simulink model "Controllo_LQ_comp"  (R2023b)
settings: Solver=VariableStepAuto  StartTime=0.0  StopTime=100  RelTol=1e-6
undefined symbols (not defined in the file): A, B, C, Comp, D, K
settings Model: Creator=alfredo  LastModifiedBy=roberto_ambrosino
settings SolverCC: AlgebraicLoopSolver=TrustRegion
settings DataIOCC: ReturnWorkspaceOutputs=off
settings DebuggingCC: UnconnectedInputMsg=warning  UnconnectedOutputMsg=warning  UnconnectedLineMsg=warning  ArithmeticOperatorsInVariantConditions=warning
settings ModelReferenceCC: EnableRefExpFcnMdlSchedulingChecks=on
settings SFSimCC: SimUseLocalCustomCode=off  CustomCodeUndefinedFunction=UseInterfaceOnly
settings RTWCC: RTWUseLocalCustomCode=off

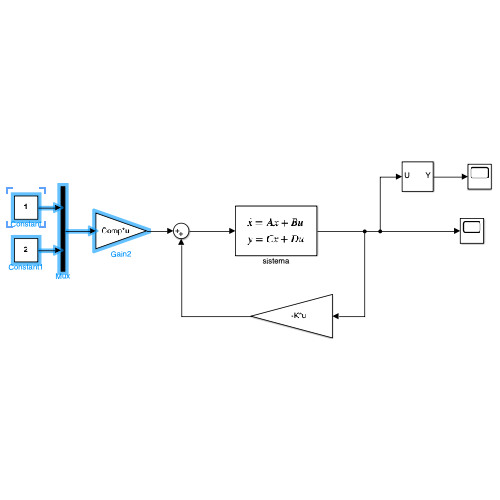
[thumbnail: Simulink's stored preview of the top-level diagram]
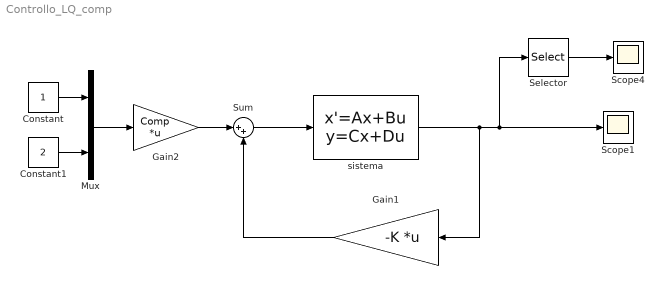
== system Controllo_LQ_comp ==
  Constant : Constant
  Constant1 : Constant  Value=2
  Gain1 : Gain  Gain=-K  Multiplication=Matrix(K*u)
  Gain2 : Gain  Gain=Comp  Multiplication=Matrix(K*u)
  Mux : Mux  Inputs=2
  Scope1 : Scope
  Scope4 : Scope
  Selector : Selector  InputPortWidth=6  IndexOptions=Index vector (dialog)  Indices=[1 5]  OutputSizes=1
  Sum : Sum  Inputs=|++
  sistema : StateSpace  A=A  B=B  C=C  D=D  InitialCondition=[1 0 1 0 1 0]
  wires:
  Sum/1 -> sistema/1
  Gain1/1 -> Sum/2
  Gain2/1 -> Sum/1
  Mux/1 -> Gain2/1
  Constant/1 -> Mux/1
  Constant1/1 -> Mux/2
  sistema/1 -> Selector/1, Scope1/1, Gain1/1
  Selector/1 -> Scope4/1
